simulink model "wmiko_xwrhtiko"  (R2022a)
settings: Solver=ode23tb  StartTime=0.0  StopTime=3  MaxStep=1e-5  RelTol=1e-3
libraries: spsRMSLib x6, spsCurrentMeasurementLib x4, spsPowerLib x2, spsVoltageMeasurementLib x2, spsSeriesRLCBranchLib x2, spsControlledVoltageSourceLib x1, simulink x1, spsSaturableTransformerLib x1, spspowerguiLib x1
settings Model: Creator=User  LastModifiedBy=User

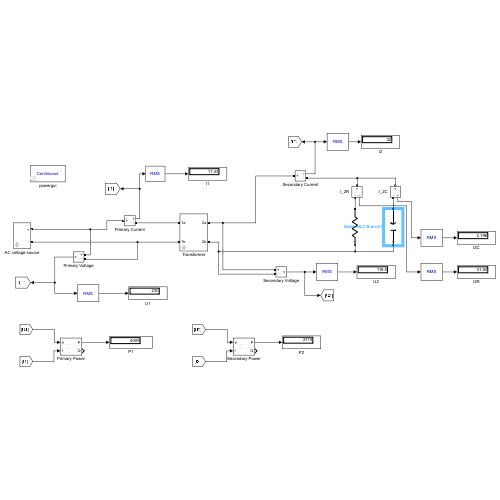
[thumbnail: Simulink's stored preview of the top-level diagram]
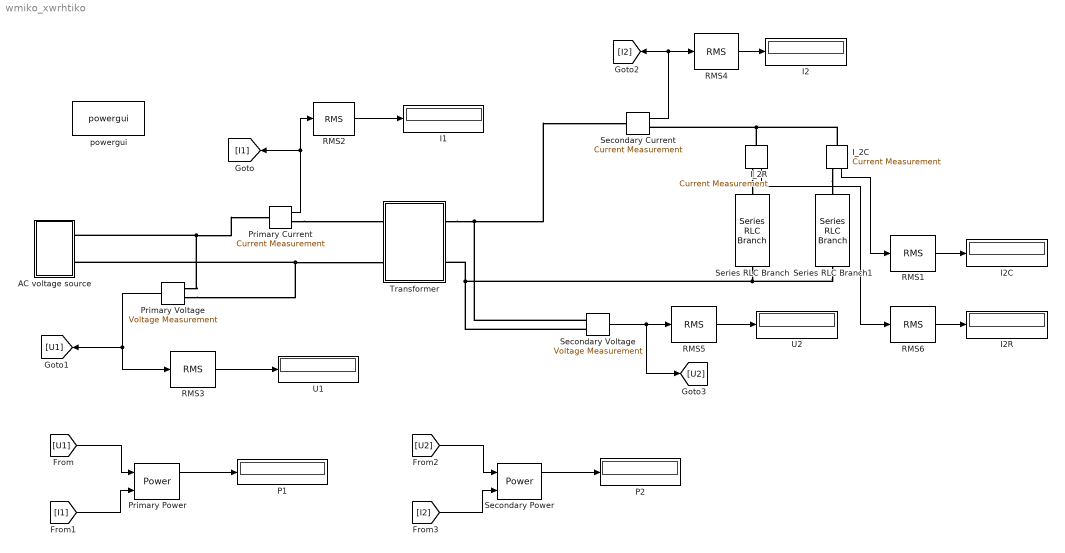
== system wmiko_xwrhtiko ==
  AC voltage source : Subsystem  mask{Vrms=230}
  I1 : Display
  I2 : Display
  I2C : Display
  I2R : Display
  I_2C : spsCurrentMeasurementLib/Current Measurement  PhasorSimulation=off  OutputType=Complex  PSBequivalent=0
  I_2R : spsCurrentMeasurementLib/Current Measurement  PhasorSimulation=off  OutputType=Complex  PSBequivalent=0
  P1 : Display
  P2 : Display
  Primary Current : spsCurrentMeasurementLib/Current Measurement  PhasorSimulation=off  OutputType=Complex  PSBequivalent=0
  Primary Power : spsPowerLib/Power  Freq=50  Vinit=[0, 0]  Iinit=[0, 0]  Ts=0
      settings: SourceProductBaseCode=PS
  Primary Voltage : spsVoltageMeasurementLib/Voltage Measurement  PhasorSimulation=off  OutputType=Complex  PSBequivalent=0
  RMS{1..6} (6 alike) : spsRMSLib/RMS  TrueRMS=on  Freq=50  RMSInit=0  Ts=0
  Secondary Current : spsCurrentMeasurementLib/Current Measurement  PhasorSimulation=off  OutputType=Complex  PSBequivalent=0
  Secondary Power : spsPowerLib/Power  Freq=50  Vinit=[0, 0]  Iinit=[0, 0]  Ts=0
      settings: SourceProductBaseCode=PS
  Secondary Voltage : spsVoltageMeasurementLib/Voltage Measurement  PhasorSimulation=off  OutputType=Complex  PSBequivalent=0
  Series RLC Branch : spsSeriesRLCBranchLib/Series RLC Branch  LConnTagsString=__new0  RConnTagsString=__new0  BranchType=R  Resistance=3.65  Inductance=1e-3  SetiL0=off  InitialCurrent=0  Capacitance=1e-6  Setx0=off  InitialVoltage=0  Measurements=None
  Series RLC Branch1 : spsSeriesRLCBranchLib/Series RLC Branch  LConnTagsString=__new0  RConnTagsString=__new0  BranchType=C  Resistance=10  Inductance=20e-3  SetiL0=off  InitialCurrent=0  Capacitance=10e-6  Setx0=off  InitialVoltage=0  Measurements=None
  Transformer : Subsystem  mask{PN=4, U1N=230, U2N=115}
      mask prompts: PN "PN (kVA)"; U1N "U1N (V)"; U2N "U2N (V)"
  U1 : Display
  U2 : Display
  powergui : spspowerguiLib/powergui  Priority=1  SimulationMode=Continuous  SampleTime=50e-6  frequency=60  Iterations=50  frequencyindice=0  Pbase=100e6  ErrMax=1e-4  UnitsV=kV  UnitsW=MW  buscounter=0  FunctionMessages=off  echomessages=off  EnableUseOfTLC=off  CurrentSourceSwitches=off  DisableSnubberDevices=off  DisableRonSwitches=off  DisableVfSwitches=off  DisplayEquations=off  AutomaticDiscreteSolvers=off  SolverType=Tustin/Backward Euler (TBE)  Interpol=off  ExternalGateDelay=off  methode=off  Ts=100  x0status=blocks  SPID=on  SwTol=0  HookPort=off  NonlinearTolerance=1e-4  nMaxIteration=100  ContinueOnMaxIteration=off  RestoreLinks=warning  ResistiveCurrentMeasurement=off  Frange=[0:2:500]  Ylog=off  Xlog=on  ShowGrid=off  save=off  variable=ZData  structure=0  ZoomFFT=off  StartTime=0.0  cycles=1  DisplayStyle=1  fundamental=60  FreqAxis=off  MaxFrequency=1000  frequencyindicesteady=1  RmsSteady=1  display=off
  wires:
  RMS3/1 -> U1/1
  [I2] -> Secondary Power/2
  [U1] -> Primary Power/1
  RMS5/1 -> U2/1
  [I1] -> Primary Power/2
  Primary Current/1 -> RMS2/1, [I1]
  [U2] -> Secondary Power/1
  RMS4/1 -> I2/1
  Secondary Current/1 -> [I2], RMS4/1
  RMS2/1 -> I1/1
  Secondary Voltage/1 -> [U2], RMS5/1
  I_2C/1 -> RMS1/1
  Primary Power/1 -> P1/1
  I_2R/1 -> RMS6/1
  Primary Voltage/1 -> [U1], RMS3/1
  RMS6/1 -> I2R/1
  Secondary Power/1 -> P2/1
  RMS1/1 -> I2C/1
  connections:
  Series RLC Branch/LConn1 -- Secondary Voltage/LConn2 -- Transformer/RConn2 -- Series RLC Branch1/LConn1
  Secondary Voltage/LConn1 -- Secondary Current/LConn1 -- Transformer/RConn1
  AC voltage source/RConn1 -- Primary Voltage/LConn1 -- Primary Current/LConn1
  Secondary Current/RConn1 -- I_2R/LConn1 -- I_2C/LConn1
  AC voltage source/RConn2 -- Transformer/LConn2 -- Primary Voltage/LConn2
  I_2C/RConn1 -- Series RLC Branch1/RConn1
  Primary Current/RConn1 -- Transformer/LConn1
  I_2R/RConn1 -- Series RLC Branch/RConn1

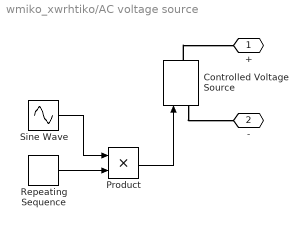
== system wmiko_xwrhtiko/AC voltage source ==
  Controlled Voltage Source : spsControlledVoltageSourceLib/Controlled Voltage Source  Initialize=on  Source_Type=AC  Amplitude=0  Phase=0  Frequency=50  Measurements=Voltage
  Product : Product
  Repeating Sequence : simulink/Sources/Repeating Sequence  rep_seq_t=[0 0.5 1000]  rep_seq_y=[0 Vrms Vrms]
  Sine Wave : Sin  Amplitude=sqrt(2)  Frequency=100*pi  SampleTime=0
  + : PMIOPort  Side=Right
  - : PMIOPort  Port=2  Side=Right
  wires:
  Product/1 -> Controlled Voltage Source/1
  Sine Wave/1 -> Product/1
  Repeating Sequence/1 -> Product/2
  connections:
  Controlled Voltage Source/LConn1 -- -/RConn1
  Controlled Voltage Source/RConn1 -- +/RConn1

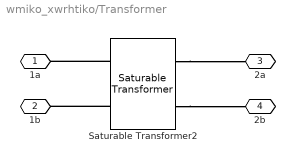
== system wmiko_xwrhtiko/Transformer ==
  Saturable Transformer2 : spsSaturableTransformerLib/Saturable Transformer  ThreeWindings=off  Hysteresis=off  DataFile='hysteresis.mat'  Measurements=None  UNITS=pu  NominalPower=[4e3 50]  Winding1=[230 0.022273 0.015903]  Winding2=[122 0.024298 0.019083]  Winding3=[3.15e+05 0.00245 0.098001]  Saturation=[0 0;0.031714 0.76205;0.037813 0.86926;0.045538 0.94653;0.060175 1.0141;0.080911 1.0624;0.14637 1.159]  CoreLoss=35.539  BreakLoop=off  DiscreteSolver=Trapezoidal iterative  DataType=off  InitialFlux=0  TransfoNumber=1
      settings: SourceProductBaseCode=PS
  1a : PMIOPort  Side=Left
  1b : PMIOPort  Port=2  Side=Left
  2a : PMIOPort  Port=3  Side=Right
  2b : PMIOPort  Port=4  Side=Right
  connections:
  Saturable Transformer2/RConn2 -- 2b/RConn1
  Saturable Transformer2/LConn1 -- 1a/RConn1
  Saturable Transformer2/RConn1 -- 2a/RConn1
  Saturable Transformer2/LConn2 -- 1b/RConn1
